simulink model "PID_regulator"  (R2021a)
settings: Solver=ode23  StartTime=0.0  StopTime=1  RelTol=1e-5
values from neighbouring files (symbols this model uses):
  Ce = 0.96    [BCMotor_params.mat]    (also in p_3_6.m = 0.058; paragraph 3_3_1.mat = 0.153; paragraph 3_3_2.mat = 0.153; paragraph 3_3_3.mat = 0.153)
  Cm = 1.85    [BCMotor_params.mat]    (also in p_3_6.m = 0.057; paragraph 3_3_1.mat = 0.156; paragraph 3_3_2.mat = 0.156; paragraph 3_3_3.mat = 0.156)
  J = 2.02e-05    [BCMotor_params.mat]    (also in p_3_6.m = 8.4e-05; paragraph 3_3_1.mat = 0.000122; paragraph 3_3_2.mat = 0.000122; paragraph 3_3_3.mat = 0.000122)
  Kd = 0    [paragraph 3_3_1.mat]    (also in paragraph 3_3_2.mat; paragraph 3_3_3.mat = 0.00180285967315; paragraph_3_6.mat = 0.0307302532304; paragraph_3_7.mat = 0.111880875618)
  Ki = 1.99103110405    [paragraph 3_3_1.mat]    (also in paragraph 3_3_2.mat = 19.7366061918; paragraph 3_3_3.mat = 0.0115578770167; paragraph_3_6.mat = 55.8570094609; paragraph_3_7.mat = 4.13901329726)
  Kp = 0    [paragraph 3_3_1.mat]    (also in paragraph 3_3_2.mat = 0.0345995362261; paragraph 3_3_3.mat = 0.327575289447; paragraph_3_6.mat = 3.29765305109; paragraph_3_7.mat = 4.54282647153)
  Ly = 0.86e-3    (= 0.00086)    [p_3_6.m]    (also in paragraph 3_3_1.mat = 0.0001; paragraph 3_3_2.mat = 0.0001; paragraph 3_3_3.mat = 0.0001; paragraph_3 5.mat = 0.0001)
  Ry = 0.71    [p_3_6.m]    (also in paragraph 3_3_1.mat = 0.34; paragraph 3_3_2.mat = 0.34; paragraph 3_3_3.mat = 0.34; paragraph_3 5.mat = 0.34)
libraries: checkpacklib x6, pid_lib x6
settings Model: Creator=slagt  LastModifiedBy=slagt

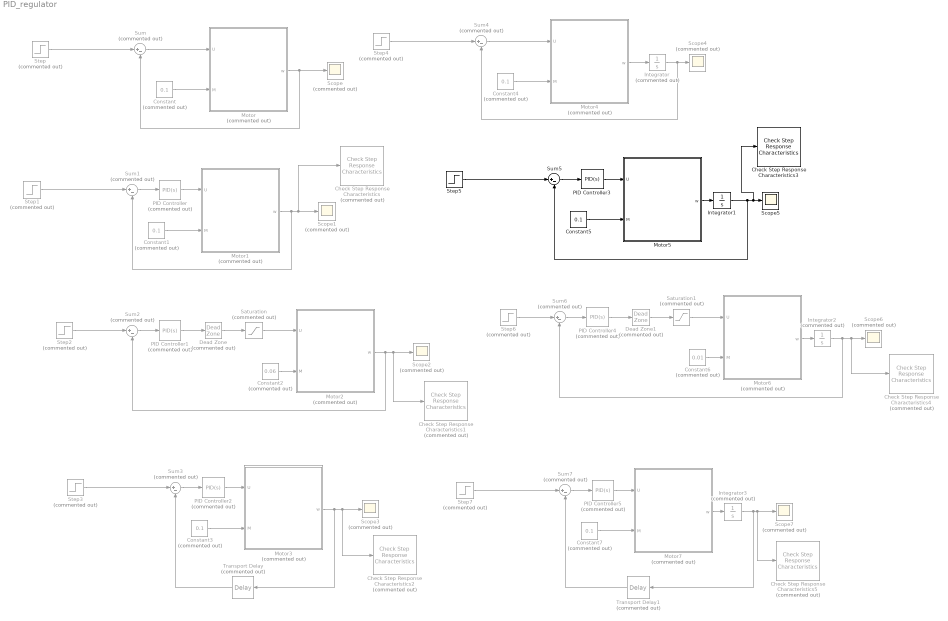
== system PID_regulator ==
  Check Step Response Characteristics : checkpacklib/Check Step Response  Characteristics  Commented=on  InstantiateOnLoad=on  enabled=on  stopWhenAssertionFail=off  export=off  ViewDlgPos=[1 1 1253.14285714286 968]  OpenViewOnLoad=off  LaunchViewOnOpen=off  TimeUnits=seconds  EnableStepResponseBound=on  InitialValue=0  FinalValue=1  StepTime=0  RiseTime=5  PercentRise=80  SettlingTime=7  PercentSettling=1  PercentOvershoot=10  PercentUndershoot=1
      settings: SourceProductBaseCode=CT,ID,MT,SO
  Check Step Response Characteristics{1..2,4..5} (4 alike) : checkpacklib/Check Step Response  Characteristics  Commented=on  InstantiateOnLoad=on  enabled=on  stopWhenAssertionFail=off  export=off  ViewDlgPos=[]  OpenViewOnLoad=off  LaunchViewOnOpen=off  TimeUnits=seconds  EnableStepResponseBound=on  InitialValue=0  FinalValue=1  StepTime=0  RiseTime=5  PercentRise=80  SettlingTime=7  PercentSettling=1  PercentOvershoot=10  PercentUndershoot=1
      settings: SourceProductBaseCode=CT,ID,MT,SO
  Check Step Response Characteristics3 : checkpacklib/Check Step Response  Characteristics  InstantiateOnLoad=on  enabled=on  stopWhenAssertionFail=off  export=off  ViewDlgPos=[1 1 1253.14285714286 968]  OpenViewOnLoad=off  LaunchViewOnOpen=off  TimeUnits=seconds  EnableStepResponseBound=on  InitialValue=0  FinalValue=1  StepTime=0  RiseTime=5  PercentRise=80  SettlingTime=7  PercentSettling=1  PercentOvershoot=10  PercentUndershoot=1
      settings: SourceProductBaseCode=CT,ID,MT,SO
  Constant{,1,3..4,7} (5 alike) : Constant  Commented=on  Value=0.1
  Constant2 : Constant  Commented=on  Value=0.06
  Constant5 : Constant  Value=0.1
  Constant6 : Constant  Commented=on  Value=0.01
  Dead Zone : DeadZone  Commented=on  LowerValue=-0.8  UpperValue=0.8  SaturateOnIntegerOverflow=on
  Dead Zone1 : DeadZone  Commented=on  LowerValue=-0.8  UpperValue=0.8  SaturateOnIntegerOverflow=on
  Integrator : Integrator  Commented=on
  Integrator1 : Integrator
  Integrator2 : Integrator  Commented=on
  Integrator3 : Integrator  Commented=on
  Motor : Subsystem  Commented=on
  Motor1 : Subsystem  Commented=on
  Motor2 : Subsystem  Commented=on
  Motor3 : Subsystem  Commented=on
  Motor4 : Subsystem  Commented=on
  Motor5 : Subsystem
  Motor6 : Subsystem  Commented=on
  Motor7 : Subsystem  Commented=on
  PID Controller : pid_lib/PID Controller  Commented=on  Controller=PID  Form=Parallel  TimeDomain=Continuous-time  UseExternalTs=off  SampleTime=-1  IntegratorMethod=Forward Euler  FilterMethod=Forward Euler  ControllerParametersSource=internal  P=Kp  I=Ki  D=Kd  UseFilter=on  N=100  TunerSelectOption=Frequency Response Based  InitialConditionSource=internal  InitialConditionForIntegrator=0  InitialConditionForFilter=0  DifferentiatorICPrevScaledInput=0  ExternalReset=none  TrackingMode=off  Kt=1  LimitOutput=off  SatLimitsSource=internal  UpperSaturationLimit=inf  LowerSaturationLimit=-inf  LinearizeAsGain=on  AntiWindupMode=none  Kb=1  POutMin=[]  POutMax=[]  IOutMin=[]  IOutMax=[]  DOutMin=[]  DOutMax=[]  NOutMin=[]  NOutMax=[]  SumOutMin=[]  SumOutMax=[]  SaturationOutMin=[]  SaturationOutMax=[]  PParamMin=[]  PParamMax=[]  IParamMin=[]  IParamMax=[]  DParamMin=[]  DParamMax=[]  NParamMin=[]  NParamMax=[]  KbParamMin=[]  KbParamMax=[]  KtParamMin=[]  KtParamMax=[]  KbOutMin=[]  KbOutMax=[]  KtOutMin=[]  KtOutMax=[]  IntegratorOutMin=[]  IntegratorOutMax=[]  FilterOutMin=[]  FilterOutMax=[]  SumI1OutMin=[]  SumI1OutMax=[]  SumI2OutMin=[]  SumI2OutMax=[]  SumI3OutMin=[]  SumI3OutMax=[]  SumI4OutMin=[]  SumI4OutMax=[]  SumDOutMin=[]  SumDOutMax=[]  DifferentiatorOutMin=[]  DifferentiatorOutMax=[]  FilterDiffOutCoefMin=[]  FilterDiffOutCoefMax=[]  ReciprocalOutMin=[]  ReciprocalOutMax=[]  SumDenOutMin=[]  SumDenOutMax=[]  SumNumOutMin=[]  SumNumOutMax=[]  DivideOutMin=[]  DivideOutMax=[]  UdiffTsProdOutMin=[]  UdiffTsProdOutMax=[]  NTsProdOutMin=[]  NTsProdOutMax=[]  UintegralTsProdOutMin=[]  UintegralTsProdOutMax=[]  UngainTsProdOutMin=[]  UngainTsProdOutMax=[]  IntegratorContinuousStateAttributes=''  IntegratorStateMustResolveToSignalObject=off  IntegratorRTWStateStorageClass=Auto  FilterContinuousStateAttributes=''  FilterStateMustResolveToSignalObject=off  FilterRTWStateStorageClass=Auto  ParallelPVariant=InternalParameters  IdealPVariant=Disabled  IVariant=InternalParameters  DVariant=InternalParameters  IntegratorVariant=Continuous  SatVariant=Disabled  AWVariant=Passthrough  PCopyVariant=Disabled  TRVariant=Disabled  FdbkBlocksVariant=Forward  IdealPFdbkVariant=Disabled  SatFdbkVariant=Disabled  DerivativeFilterVariant=ContFilter  NVariant=InternalParameters  NCopyVariant=Disabled  FilterICVariant=InternalICsFilter  IntegratorICVariant=InternalICs  ExternalResetVariant=Disabled  TRSumVariant=Passthrough  SumFdbkVariant=Disabled  SumVariant=Sum_PID  TsampFilterVariant=InternalTs  TsampNgainVariant=Passthrough  TsampIntegralVariant=Passthrough  ExternalSaturationOutDataTypeStr=Inherit: Same as second input
  PID Controller1 : pid_lib/PID Controller  Commented=on  Controller=PID  Form=Parallel  TimeDomain=Continuous-time  UseExternalTs=off  SampleTime=-1  IntegratorMethod=Forward Euler  FilterMethod=Forward Euler  ControllerParametersSource=internal  P=Kp  I=Ki  D=Kd  UseFilter=on  N=100  TunerSelectOption=Transfer Function Based (PID Tuner App)  InitialConditionSource=internal  InitialConditionForIntegrator=0  InitialConditionForFilter=0  DifferentiatorICPrevScaledInput=0  ExternalReset=none  TrackingMode=off  Kt=1  LimitOutput=off  SatLimitsSource=internal  UpperSaturationLimit=inf  LowerSaturationLimit=-inf  LinearizeAsGain=on  AntiWindupMode=none  Kb=1  POutMin=[]  POutMax=[]  IOutMin=[]  IOutMax=[]  DOutMin=[]  DOutMax=[]  NOutMin=[]  NOutMax=[]  SumOutMin=[]  SumOutMax=[]  SaturationOutMin=[]  SaturationOutMax=[]  PParamMin=[]  PParamMax=[]  IParamMin=[]  IParamMax=[]  DParamMin=[]  DParamMax=[]  NParamMin=[]  NParamMax=[]  KbParamMin=[]  KbParamMax=[]  KtParamMin=[]  KtParamMax=[]  KbOutMin=[]  KbOutMax=[]  KtOutMin=[]  KtOutMax=[]  IntegratorOutMin=[]  IntegratorOutMax=[]  FilterOutMin=[]  FilterOutMax=[]  SumI1OutMin=[]  SumI1OutMax=[]  SumI2OutMin=[]  SumI2OutMax=[]  SumI3OutMin=[]  SumI3OutMax=[]  SumI4OutMin=[]  SumI4OutMax=[]  SumDOutMin=[]  SumDOutMax=[]  DifferentiatorOutMin=[]  DifferentiatorOutMax=[]  FilterDiffOutCoefMin=[]  FilterDiffOutCoefMax=[]  ReciprocalOutMin=[]  ReciprocalOutMax=[]  SumDenOutMin=[]  SumDenOutMax=[]  SumNumOutMin=[]  SumNumOutMax=[]  DivideOutMin=[]  DivideOutMax=[]  UdiffTsProdOutMin=[]  UdiffTsProdOutMax=[]  NTsProdOutMin=[]  NTsProdOutMax=[]  UintegralTsProdOutMin=[]  UintegralTsProdOutMax=[]  UngainTsProdOutMin=[]  UngainTsProdOutMax=[]  IntegratorContinuousStateAttributes=''  IntegratorStateMustResolveToSignalObject=off  IntegratorRTWStateStorageClass=Auto  FilterContinuousStateAttributes=''  FilterStateMustResolveToSignalObject=off  FilterRTWStateStorageClass=Auto  ParallelPVariant=InternalParameters  IdealPVariant=Disabled  IVariant=InternalParameters  DVariant=InternalParameters  IntegratorVariant=Continuous  SatVariant=Disabled  AWVariant=Passthrough  PCopyVariant=Disabled  TRVariant=Disabled  FdbkBlocksVariant=Forward  IdealPFdbkVariant=Disabled  SatFdbkVariant=Disabled  DerivativeFilterVariant=ContFilter  NVariant=InternalParameters  NCopyVariant=Disabled  FilterICVariant=InternalICsFilter  IntegratorICVariant=InternalICs  ExternalResetVariant=Disabled  TRSumVariant=Passthrough  SumFdbkVariant=Disabled  SumVariant=Sum_PID  TsampFilterVariant=InternalTs  TsampNgainVariant=Passthrough  TsampIntegralVariant=Passthrough  ExternalSaturationOutDataTypeStr=Inherit: Same as second input
  PID Controller2 : pid_lib/PID Controller  Commented=on  Controller=PID  Form=Parallel  TimeDomain=Continuous-time  UseExternalTs=off  SampleTime=-1  IntegratorMethod=Forward Euler  FilterMethod=Forward Euler  ControllerParametersSource=internal  P=Kp  I=Ki  D=Kd  UseFilter=on  N=100  TunerSelectOption=Transfer Function Based (PID Tuner App)  InitialConditionSource=internal  InitialConditionForIntegrator=0  InitialConditionForFilter=0  DifferentiatorICPrevScaledInput=0  ExternalReset=none  TrackingMode=off  Kt=1  LimitOutput=off  SatLimitsSource=internal  UpperSaturationLimit=inf  LowerSaturationLimit=-inf  LinearizeAsGain=on  AntiWindupMode=none  Kb=1  POutMin=[]  POutMax=[]  IOutMin=[]  IOutMax=[]  DOutMin=[]  DOutMax=[]  NOutMin=[]  NOutMax=[]  SumOutMin=[]  SumOutMax=[]  SaturationOutMin=[]  SaturationOutMax=[]  PParamMin=[]  PParamMax=[]  IParamMin=[]  IParamMax=[]  DParamMin=[]  DParamMax=[]  NParamMin=[]  NParamMax=[]  KbParamMin=[]  KbParamMax=[]  KtParamMin=[]  KtParamMax=[]  KbOutMin=[]  KbOutMax=[]  KtOutMin=[]  KtOutMax=[]  IntegratorOutMin=[]  IntegratorOutMax=[]  FilterOutMin=[]  FilterOutMax=[]  SumI1OutMin=[]  SumI1OutMax=[]  SumI2OutMin=[]  SumI2OutMax=[]  SumI3OutMin=[]  SumI3OutMax=[]  SumI4OutMin=[]  SumI4OutMax=[]  SumDOutMin=[]  SumDOutMax=[]  DifferentiatorOutMin=[]  DifferentiatorOutMax=[]  FilterDiffOutCoefMin=[]  FilterDiffOutCoefMax=[]  ReciprocalOutMin=[]  ReciprocalOutMax=[]  SumDenOutMin=[]  SumDenOutMax=[]  SumNumOutMin=[]  SumNumOutMax=[]  DivideOutMin=[]  DivideOutMax=[]  UdiffTsProdOutMin=[]  UdiffTsProdOutMax=[]  NTsProdOutMin=[]  NTsProdOutMax=[]  UintegralTsProdOutMin=[]  UintegralTsProdOutMax=[]  UngainTsProdOutMin=[]  UngainTsProdOutMax=[]  IntegratorContinuousStateAttributes=''  IntegratorStateMustResolveToSignalObject=off  IntegratorRTWStateStorageClass=Auto  FilterContinuousStateAttributes=''  FilterStateMustResolveToSignalObject=off  FilterRTWStateStorageClass=Auto  ParallelPVariant=InternalParameters  IdealPVariant=Disabled  IVariant=InternalParameters  DVariant=InternalParameters  IntegratorVariant=Continuous  SatVariant=Disabled  AWVariant=Passthrough  PCopyVariant=Disabled  TRVariant=Disabled  FdbkBlocksVariant=Forward  IdealPFdbkVariant=Disabled  SatFdbkVariant=Disabled  DerivativeFilterVariant=ContFilter  NVariant=InternalParameters  NCopyVariant=Disabled  FilterICVariant=InternalICsFilter  IntegratorICVariant=InternalICs  ExternalResetVariant=Disabled  TRSumVariant=Passthrough  SumFdbkVariant=Disabled  SumVariant=Sum_PID  TsampFilterVariant=InternalTs  TsampNgainVariant=Passthrough  TsampIntegralVariant=Passthrough  ExternalSaturationOutDataTypeStr=Inherit: Same as second input
  PID Controller3 : pid_lib/PID Controller  Controller=PID  Form=Parallel  TimeDomain=Continuous-time  UseExternalTs=off  SampleTime=-1  IntegratorMethod=Forward Euler  FilterMethod=Forward Euler  ControllerParametersSource=internal  P=Kp  I=Ki  D=Kd  UseFilter=on  N=100  TunerSelectOption=Transfer Function Based (PID Tuner App)  InitialConditionSource=internal  InitialConditionForIntegrator=0  InitialConditionForFilter=0  DifferentiatorICPrevScaledInput=0  ExternalReset=none  TrackingMode=off  Kt=1  LimitOutput=off  SatLimitsSource=internal  UpperSaturationLimit=inf  LowerSaturationLimit=-inf  LinearizeAsGain=on  AntiWindupMode=none  Kb=1  POutMin=[]  POutMax=[]  IOutMin=[]  IOutMax=[]  DOutMin=[]  DOutMax=[]  NOutMin=[]  NOutMax=[]  SumOutMin=[]  SumOutMax=[]  SaturationOutMin=[]  SaturationOutMax=[]  PParamMin=[]  PParamMax=[]  IParamMin=[]  IParamMax=[]  DParamMin=[]  DParamMax=[]  NParamMin=[]  NParamMax=[]  KbParamMin=[]  KbParamMax=[]  KtParamMin=[]  KtParamMax=[]  KbOutMin=[]  KbOutMax=[]  KtOutMin=[]  KtOutMax=[]  IntegratorOutMin=[]  IntegratorOutMax=[]  FilterOutMin=[]  FilterOutMax=[]  SumI1OutMin=[]  SumI1OutMax=[]  SumI2OutMin=[]  SumI2OutMax=[]  SumI3OutMin=[]  SumI3OutMax=[]  SumI4OutMin=[]  SumI4OutMax=[]  SumDOutMin=[]  SumDOutMax=[]  DifferentiatorOutMin=[]  DifferentiatorOutMax=[]  FilterDiffOutCoefMin=[]  FilterDiffOutCoefMax=[]  ReciprocalOutMin=[]  ReciprocalOutMax=[]  SumDenOutMin=[]  SumDenOutMax=[]  SumNumOutMin=[]  SumNumOutMax=[]  DivideOutMin=[]  DivideOutMax=[]  UdiffTsProdOutMin=[]  UdiffTsProdOutMax=[]  NTsProdOutMin=[]  NTsProdOutMax=[]  UintegralTsProdOutMin=[]  UintegralTsProdOutMax=[]  UngainTsProdOutMin=[]  UngainTsProdOutMax=[]  IntegratorContinuousStateAttributes=''  IntegratorStateMustResolveToSignalObject=off  IntegratorRTWStateStorageClass=Auto  FilterContinuousStateAttributes=''  FilterStateMustResolveToSignalObject=off  FilterRTWStateStorageClass=Auto  ParallelPVariant=InternalParameters  IdealPVariant=Disabled  IVariant=InternalParameters  DVariant=InternalParameters  IntegratorVariant=Continuous  SatVariant=Disabled  AWVariant=Passthrough  PCopyVariant=Disabled  TRVariant=Disabled  FdbkBlocksVariant=Forward  IdealPFdbkVariant=Disabled  SatFdbkVariant=Disabled  DerivativeFilterVariant=ContFilter  NVariant=InternalParameters  NCopyVariant=Disabled  FilterICVariant=InternalICsFilter  IntegratorICVariant=InternalICs  ExternalResetVariant=Disabled  TRSumVariant=Passthrough  SumFdbkVariant=Disabled  SumVariant=Sum_PID  TsampFilterVariant=InternalTs  TsampNgainVariant=Passthrough  TsampIntegralVariant=Passthrough  ExternalSaturationOutDataTypeStr=Inherit: Same as second input
  PID Controller4 : pid_lib/PID Controller  Commented=on  Controller=PID  Form=Parallel  TimeDomain=Continuous-time  UseExternalTs=off  SampleTime=-1  IntegratorMethod=Forward Euler  FilterMethod=Forward Euler  ControllerParametersSource=internal  P=Kp  I=Ki  D=Kd  UseFilter=on  N=12179.3371375547  TunerSelectOption=Transfer Function Based (PID Tuner App)  InitialConditionSource=internal  InitialConditionForIntegrator=0  InitialConditionForFilter=0  DifferentiatorICPrevScaledInput=0  ExternalReset=none  TrackingMode=off  Kt=1  LimitOutput=off  SatLimitsSource=internal  UpperSaturationLimit=inf  LowerSaturationLimit=-inf  LinearizeAsGain=on  AntiWindupMode=none  Kb=1  POutMin=[]  POutMax=[]  IOutMin=[]  IOutMax=[]  DOutMin=[]  DOutMax=[]  NOutMin=[]  NOutMax=[]  SumOutMin=[]  SumOutMax=[]  SaturationOutMin=[]  SaturationOutMax=[]  PParamMin=[]  PParamMax=[]  IParamMin=[]  IParamMax=[]  DParamMin=[]  DParamMax=[]  NParamMin=[]  NParamMax=[]  KbParamMin=[]  KbParamMax=[]  KtParamMin=[]  KtParamMax=[]  KbOutMin=[]  KbOutMax=[]  KtOutMin=[]  KtOutMax=[]  IntegratorOutMin=[]  IntegratorOutMax=[]  FilterOutMin=[]  FilterOutMax=[]  SumI1OutMin=[]  SumI1OutMax=[]  SumI2OutMin=[]  SumI2OutMax=[]  SumI3OutMin=[]  SumI3OutMax=[]  SumI4OutMin=[]  SumI4OutMax=[]  SumDOutMin=[]  SumDOutMax=[]  DifferentiatorOutMin=[]  DifferentiatorOutMax=[]  FilterDiffOutCoefMin=[]  FilterDiffOutCoefMax=[]  ReciprocalOutMin=[]  ReciprocalOutMax=[]  SumDenOutMin=[]  SumDenOutMax=[]  SumNumOutMin=[]  SumNumOutMax=[]  DivideOutMin=[]  DivideOutMax=[]  UdiffTsProdOutMin=[]  UdiffTsProdOutMax=[]  NTsProdOutMin=[]  NTsProdOutMax=[]  UintegralTsProdOutMin=[]  UintegralTsProdOutMax=[]  UngainTsProdOutMin=[]  UngainTsProdOutMax=[]  IntegratorContinuousStateAttributes=''  IntegratorStateMustResolveToSignalObject=off  IntegratorRTWStateStorageClass=Auto  FilterContinuousStateAttributes=''  FilterStateMustResolveToSignalObject=off  FilterRTWStateStorageClass=Auto  ParallelPVariant=InternalParameters  IdealPVariant=Disabled  IVariant=InternalParameters  DVariant=InternalParameters  IntegratorVariant=Continuous  SatVariant=Disabled  AWVariant=Passthrough  PCopyVariant=Disabled  TRVariant=Disabled  FdbkBlocksVariant=Forward  IdealPFdbkVariant=Disabled  SatFdbkVariant=Disabled  DerivativeFilterVariant=ContFilter  NVariant=InternalParameters  NCopyVariant=Disabled  FilterICVariant=InternalICsFilter  IntegratorICVariant=InternalICs  ExternalResetVariant=Disabled  TRSumVariant=Passthrough  SumFdbkVariant=Disabled  SumVariant=Sum_PID  TsampFilterVariant=InternalTs  TsampNgainVariant=Passthrough  TsampIntegralVariant=Passthrough  ExternalSaturationOutDataTypeStr=Inherit: Same as second input
  PID Controller5 : pid_lib/PID Controller  Commented=on  Controller=PID  Form=Parallel  TimeDomain=Continuous-time  UseExternalTs=off  SampleTime=-1  IntegratorMethod=Forward Euler  FilterMethod=Forward Euler  ControllerParametersSource=internal  P=Kp  I=Ki  D=Kd  UseFilter=on  N=0.475761307334443  TunerSelectOption=Transfer Function Based (PID Tuner App)  InitialConditionSource=internal  InitialConditionForIntegrator=0  InitialConditionForFilter=0  DifferentiatorICPrevScaledInput=0  ExternalReset=none  TrackingMode=off  Kt=1  LimitOutput=off  SatLimitsSource=internal  UpperSaturationLimit=inf  LowerSaturationLimit=-inf  LinearizeAsGain=on  AntiWindupMode=none  Kb=1  POutMin=[]  POutMax=[]  IOutMin=[]  IOutMax=[]  DOutMin=[]  DOutMax=[]  NOutMin=[]  NOutMax=[]  SumOutMin=[]  SumOutMax=[]  SaturationOutMin=[]  SaturationOutMax=[]  PParamMin=[]  PParamMax=[]  IParamMin=[]  IParamMax=[]  DParamMin=[]  DParamMax=[]  NParamMin=[]  NParamMax=[]  KbParamMin=[]  KbParamMax=[]  KtParamMin=[]  KtParamMax=[]  KbOutMin=[]  KbOutMax=[]  KtOutMin=[]  KtOutMax=[]  IntegratorOutMin=[]  IntegratorOutMax=[]  FilterOutMin=[]  FilterOutMax=[]  SumI1OutMin=[]  SumI1OutMax=[]  SumI2OutMin=[]  SumI2OutMax=[]  SumI3OutMin=[]  SumI3OutMax=[]  SumI4OutMin=[]  SumI4OutMax=[]  SumDOutMin=[]  SumDOutMax=[]  DifferentiatorOutMin=[]  DifferentiatorOutMax=[]  FilterDiffOutCoefMin=[]  FilterDiffOutCoefMax=[]  ReciprocalOutMin=[]  ReciprocalOutMax=[]  SumDenOutMin=[]  SumDenOutMax=[]  SumNumOutMin=[]  SumNumOutMax=[]  DivideOutMin=[]  DivideOutMax=[]  UdiffTsProdOutMin=[]  UdiffTsProdOutMax=[]  NTsProdOutMin=[]  NTsProdOutMax=[]  UintegralTsProdOutMin=[]  UintegralTsProdOutMax=[]  UngainTsProdOutMin=[]  UngainTsProdOutMax=[]  IntegratorContinuousStateAttributes=''  IntegratorStateMustResolveToSignalObject=off  IntegratorRTWStateStorageClass=Auto  FilterContinuousStateAttributes=''  FilterStateMustResolveToSignalObject=off  FilterRTWStateStorageClass=Auto  ParallelPVariant=InternalParameters  IdealPVariant=Disabled  IVariant=InternalParameters  DVariant=InternalParameters  IntegratorVariant=Continuous  SatVariant=Disabled  AWVariant=Passthrough  PCopyVariant=Disabled  TRVariant=Disabled  FdbkBlocksVariant=Forward  IdealPFdbkVariant=Disabled  SatFdbkVariant=Disabled  DerivativeFilterVariant=ContFilter  NVariant=InternalParameters  NCopyVariant=Disabled  FilterICVariant=InternalICsFilter  IntegratorICVariant=InternalICs  ExternalResetVariant=Disabled  TRSumVariant=Passthrough  SumFdbkVariant=Disabled  SumVariant=Sum_PID  TsampFilterVariant=InternalTs  TsampNgainVariant=Passthrough  TsampIntegralVariant=Passthrough  ExternalSaturationOutDataTypeStr=Inherit: Same as second input
  Saturation : Saturate  Commented=on  UpperLimit=0.15  LowerLimit=-0.15
  Saturation1 : Saturate  Commented=on  UpperLimit=0.15  LowerLimit=-0.15
  Scope{,1..4,6..7} (7 alike) : Scope  Commented=on
  Scope5 : Scope
  Step{,1..4,6..7} (7 alike) : Step  Commented=on  Time=0  SampleTime=0
  Step5 : Step  Time=0  SampleTime=0
  Sum{,1..4,6..7} (7 alike) : Sum  Commented=on  Inputs=|+-
  Sum5 : Sum  Inputs=|+-
  Transport Delay : TransportDelay  Commented=on  DelayTime=0.5
  Transport Delay1 : TransportDelay  Commented=on  DelayTime=0.5
  wires:
  Motor/1(w) -> Sum/2, Scope/1
  Constant/1 -> Motor/2(M)
  Step/1 -> Sum/1
  Sum/1 -> Motor/1(U)
  Step1/1 -> Sum1/1
  Constant1/1 -> Motor1/2(M)
  Motor1/1(w) -> Check Step Response Characteristics/1, Scope1/1, Sum1/2
  Constant2/1 -> Motor2/2(M)
  Motor2/1(w) -> Check Step Response Characteristics1/1, Scope2/1, Sum2/2
  Step2/1 -> Sum2/1
  Sum2/1 -> PID Controller1/1
  PID Controller1/1 -> Dead Zone/1
  Dead Zone/1 -> Saturation/1
  Saturation/1 -> Motor2/1(U)
  PID Controller2/1 -> Motor3/1(U)
  Constant3/1 -> Motor3/2(M)
  Motor3/1(w) -> Check Step Response Characteristics2/1, Scope3/1, Transport Delay/1
  Step3/1 -> Sum3/1
  Sum3/1 -> PID Controller2/1
  Transport Delay/1 -> Sum3/2
  PID Controller/1 -> Motor1/1(U)
  Sum1/1 -> PID Controller/1
  Constant4/1 -> Motor4/2(M)
  Sum4/1 -> Motor4/1(U)
  Step4/1 -> Sum4/1
  Constant5/1 -> Motor5/2(M)
  Step5/1 -> Sum5/1
  Sum5/1 -> PID Controller3/1
  PID Controller3/1 -> Motor5/1(U)
  Motor4/1(w) -> Integrator/1
  Integrator/1 -> Scope4/1, Sum4/2
  Motor5/1(w) -> Integrator1/1
  Integrator1/1 -> Sum5/2, Check Step Response Characteristics3/1, Scope5/1
  Saturation1/1 -> Motor6/1(U)
  Step6/1 -> Sum6/1
  Sum6/1 -> PID Controller4/1
  Dead Zone1/1 -> Saturation1/1
  Constant6/1 -> Motor6/2(M)
  PID Controller4/1 -> Dead Zone1/1
  Motor6/1(w) -> Integrator2/1
  Integrator2/1 -> Sum6/2, Check Step Response Characteristics4/1, Scope6/1
  Sum7/1 -> PID Controller5/1
  Constant7/1 -> Motor7/2(M)
  PID Controller5/1 -> Motor7/1(U)
  Step7/1 -> Sum7/1
  Transport Delay1/1 -> Sum7/2
  Motor7/1(w) -> Integrator3/1
  Integrator3/1 -> Check Step Response Characteristics5/1, Scope7/1, Transport Delay1/1

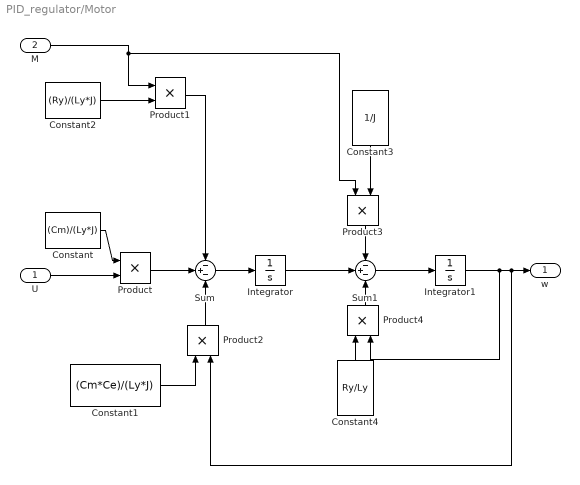
== system PID_regulator/Motor ==
  U : Inport
  M : Inport  Port=2
  Constant : Constant  Value=(Cm)/(Ly*J)
  Constant1 : Constant  Value=(Cm*Ce)/(Ly*J)
  Constant2 : Constant  Value=(Ry)/(Ly*J)
  Constant3 : Constant  Value=1/J
  Constant4 : Constant  Value=Ry/Ly
  Integrator : Integrator
  Integrator1 : Integrator
  Product{,1..4} (5 alike) : Product
  Sum : Sum  Inputs=-+-
  Sum1 : Sum  Inputs=-+-
  w : Outport
  wires:
  U/1 -> Product/2
  Product/1 -> Sum/2
  M/1 -> Product1/1, Product3/1
  Product1/1 -> Sum/1
  Constant2/1 -> Product1/2
  Product2/1 -> Sum/3
  Sum/1 -> Integrator/1
  Integrator/1 -> Sum1/2
  Sum1/1 -> Integrator1/1
  Product3/1 -> Sum1/1
  Product4/1 -> Sum1/3
  Integrator1/1 -> Product4/2, Product2/2, w/1
  Constant/1 -> Product/1
  Constant1/1 -> Product2/1
  Constant3/1 -> Product3/2
  Constant4/1 -> Product4/1

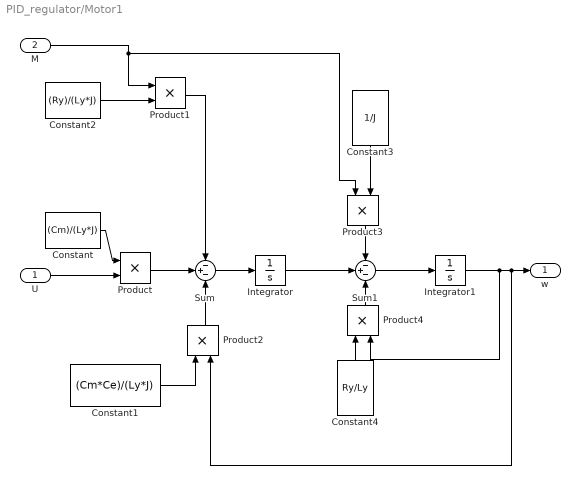
== system PID_regulator/Motor1 ==
  U : Inport
  M : Inport  Port=2
  Constant : Constant  Value=(Cm)/(Ly*J)
  Constant1 : Constant  Value=(Cm*Ce)/(Ly*J)
  Constant2 : Constant  Value=(Ry)/(Ly*J)
  Constant3 : Constant  Value=1/J
  Constant4 : Constant  Value=Ry/Ly
  Integrator : Integrator
  Integrator1 : Integrator
  Product{,1..4} (5 alike) : Product
  Sum : Sum  Inputs=-+-
  Sum1 : Sum  Inputs=-+-
  w : Outport
  wires:
  U/1 -> Product/2
  Product/1 -> Sum/2
  M/1 -> Product1/1, Product3/1
  Product1/1 -> Sum/1
  Constant2/1 -> Product1/2
  Product2/1 -> Sum/3
  Sum/1 -> Integrator/1
  Integrator/1 -> Sum1/2
  Sum1/1 -> Integrator1/1
  Product3/1 -> Sum1/1
  Product4/1 -> Sum1/3
  Integrator1/1 -> Product4/2, Product2/2, w/1
  Constant/1 -> Product/1
  Constant1/1 -> Product2/1
  Constant3/1 -> Product3/2
  Constant4/1 -> Product4/1

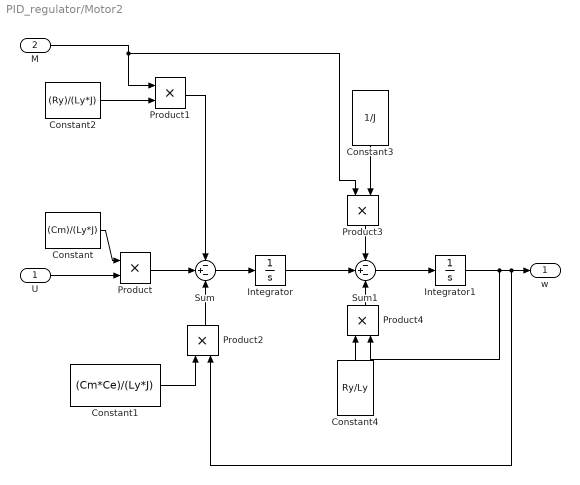
== system PID_regulator/Motor2 ==
  U : Inport
  M : Inport  Port=2
  Constant : Constant  Value=(Cm)/(Ly*J)
  Constant1 : Constant  Value=(Cm*Ce)/(Ly*J)
  Constant2 : Constant  Value=(Ry)/(Ly*J)
  Constant3 : Constant  Value=1/J
  Constant4 : Constant  Value=Ry/Ly
  Integrator : Integrator
  Integrator1 : Integrator
  Product{,1..4} (5 alike) : Product
  Sum : Sum  Inputs=-+-
  Sum1 : Sum  Inputs=-+-
  w : Outport
  wires:
  U/1 -> Product/2
  Product/1 -> Sum/2
  M/1 -> Product1/1, Product3/1
  Product1/1 -> Sum/1
  Constant2/1 -> Product1/2
  Product2/1 -> Sum/3
  Sum/1 -> Integrator/1
  Integrator/1 -> Sum1/2
  Sum1/1 -> Integrator1/1
  Product3/1 -> Sum1/1
  Product4/1 -> Sum1/3
  Integrator1/1 -> Product4/2, Product2/2, w/1
  Constant/1 -> Product/1
  Constant1/1 -> Product2/1
  Constant3/1 -> Product3/2
  Constant4/1 -> Product4/1

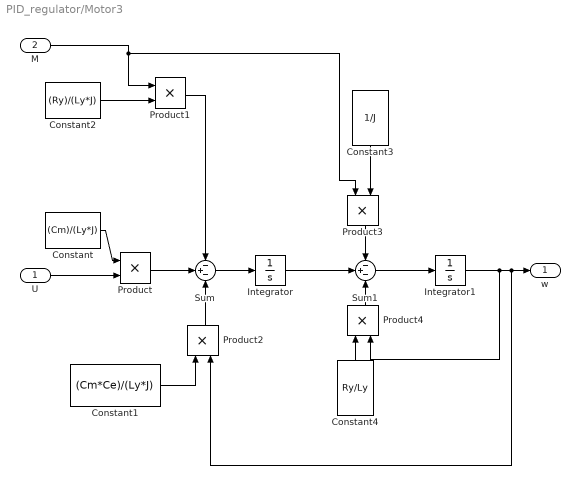
== system PID_regulator/Motor3 ==
  U : Inport
  M : Inport  Port=2
  Constant : Constant  Value=(Cm)/(Ly*J)
  Constant1 : Constant  Value=(Cm*Ce)/(Ly*J)
  Constant2 : Constant  Value=(Ry)/(Ly*J)
  Constant3 : Constant  Value=1/J
  Constant4 : Constant  Value=Ry/Ly
  Integrator : Integrator
  Integrator1 : Integrator
  Product{,1..4} (5 alike) : Product
  Sum : Sum  Inputs=-+-
  Sum1 : Sum  Inputs=-+-
  w : Outport
  wires:
  U/1 -> Product/2
  Product/1 -> Sum/2
  M/1 -> Product1/1, Product3/1
  Product1/1 -> Sum/1
  Constant2/1 -> Product1/2
  Product2/1 -> Sum/3
  Sum/1 -> Integrator/1
  Integrator/1 -> Sum1/2
  Sum1/1 -> Integrator1/1
  Product3/1 -> Sum1/1
  Product4/1 -> Sum1/3
  Integrator1/1 -> Product4/2, Product2/2, w/1
  Constant/1 -> Product/1
  Constant1/1 -> Product2/1
  Constant3/1 -> Product3/2
  Constant4/1 -> Product4/1

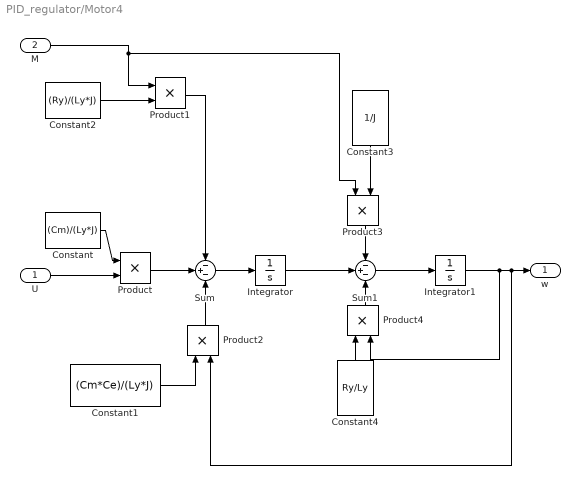
== system PID_regulator/Motor4 ==
  U : Inport
  M : Inport  Port=2
  Constant : Constant  Value=(Cm)/(Ly*J)
  Constant1 : Constant  Value=(Cm*Ce)/(Ly*J)
  Constant2 : Constant  Value=(Ry)/(Ly*J)
  Constant3 : Constant  Value=1/J
  Constant4 : Constant  Value=Ry/Ly
  Integrator : Integrator
  Integrator1 : Integrator
  Product{,1..4} (5 alike) : Product
  Sum : Sum  Inputs=-+-
  Sum1 : Sum  Inputs=-+-
  w : Outport
  wires:
  U/1 -> Product/2
  Product/1 -> Sum/2
  M/1 -> Product1/1, Product3/1
  Product1/1 -> Sum/1
  Constant2/1 -> Product1/2
  Product2/1 -> Sum/3
  Sum/1 -> Integrator/1
  Integrator/1 -> Sum1/2
  Sum1/1 -> Integrator1/1
  Product3/1 -> Sum1/1
  Product4/1 -> Sum1/3
  Integrator1/1 -> Product4/2, Product2/2, w/1
  Constant/1 -> Product/1
  Constant1/1 -> Product2/1
  Constant3/1 -> Product3/2
  Constant4/1 -> Product4/1

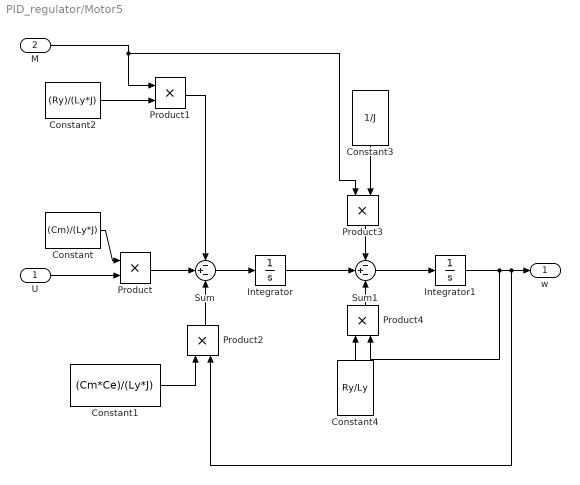
== system PID_regulator/Motor5 ==
  U : Inport
  M : Inport  Port=2
  Constant : Constant  Value=(Cm)/(Ly*J)
  Constant1 : Constant  Value=(Cm*Ce)/(Ly*J)
  Constant2 : Constant  Value=(Ry)/(Ly*J)
  Constant3 : Constant  Value=1/J
  Constant4 : Constant  Value=Ry/Ly
  Integrator : Integrator
  Integrator1 : Integrator
  Product{,1..4} (5 alike) : Product
  Sum : Sum  Inputs=-+-
  Sum1 : Sum  Inputs=-+-
  w : Outport
  wires:
  U/1 -> Product/2
  Product/1 -> Sum/2
  M/1 -> Product1/1, Product3/1
  Product1/1 -> Sum/1
  Constant2/1 -> Product1/2
  Product2/1 -> Sum/3
  Sum/1 -> Integrator/1
  Integrator/1 -> Sum1/2
  Sum1/1 -> Integrator1/1
  Product3/1 -> Sum1/1
  Product4/1 -> Sum1/3
  Integrator1/1 -> Product4/2, Product2/2, w/1
  Constant/1 -> Product/1
  Constant1/1 -> Product2/1
  Constant3/1 -> Product3/2
  Constant4/1 -> Product4/1

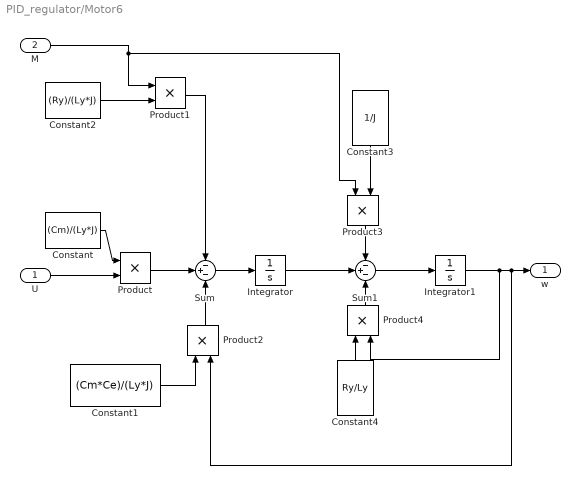
== system PID_regulator/Motor6 ==
  U : Inport
  M : Inport  Port=2
  Constant : Constant  Value=(Cm)/(Ly*J)
  Constant1 : Constant  Value=(Cm*Ce)/(Ly*J)
  Constant2 : Constant  Value=(Ry)/(Ly*J)
  Constant3 : Constant  Value=1/J
  Constant4 : Constant  Value=Ry/Ly
  Integrator : Integrator
  Integrator1 : Integrator
  Product{,1..4} (5 alike) : Product
  Sum : Sum  Inputs=-+-
  Sum1 : Sum  Inputs=-+-
  w : Outport
  wires:
  U/1 -> Product/2
  Product/1 -> Sum/2
  M/1 -> Product1/1, Product3/1
  Product1/1 -> Sum/1
  Constant2/1 -> Product1/2
  Product2/1 -> Sum/3
  Sum/1 -> Integrator/1
  Integrator/1 -> Sum1/2
  Sum1/1 -> Integrator1/1
  Product3/1 -> Sum1/1
  Product4/1 -> Sum1/3
  Integrator1/1 -> Product4/2, Product2/2, w/1
  Constant/1 -> Product/1
  Constant1/1 -> Product2/1
  Constant3/1 -> Product3/2
  Constant4/1 -> Product4/1

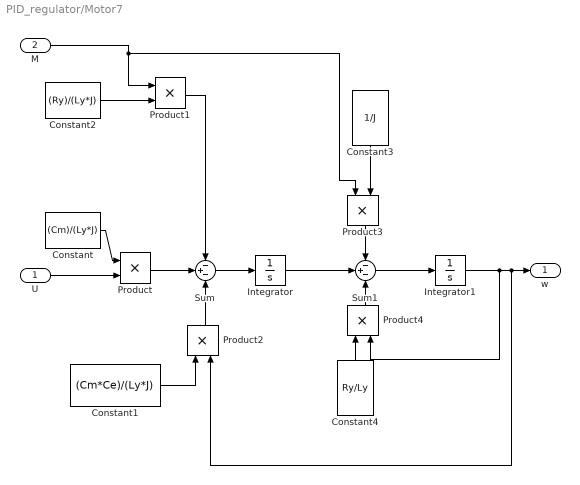
== system PID_regulator/Motor7 ==
  U : Inport
  M : Inport  Port=2
  Constant : Constant  Value=(Cm)/(Ly*J)
  Constant1 : Constant  Value=(Cm*Ce)/(Ly*J)
  Constant2 : Constant  Value=(Ry)/(Ly*J)
  Constant3 : Constant  Value=1/J
  Constant4 : Constant  Value=Ry/Ly
  Integrator : Integrator
  Integrator1 : Integrator
  Product{,1..4} (5 alike) : Product
  Sum : Sum  Inputs=-+-
  Sum1 : Sum  Inputs=-+-
  w : Outport
  wires:
  U/1 -> Product/2
  Product/1 -> Sum/2
  M/1 -> Product1/1, Product3/1
  Product1/1 -> Sum/1
  Constant2/1 -> Product1/2
  Product2/1 -> Sum/3
  Sum/1 -> Integrator/1
  Integrator/1 -> Sum1/2
  Sum1/1 -> Integrator1/1
  Product3/1 -> Sum1/1
  Product4/1 -> Sum1/3
  Integrator1/1 -> Product4/2, Product2/2, w/1
  Constant/1 -> Product/1
  Constant1/1 -> Product2/1
  Constant3/1 -> Product3/2
  Constant4/1 -> Product4/1
